simulink model "quaternion2euler"  (Simulink 10.1)
settings: Solver=VariableStepAuto  StartTime=0.0  StopTime=10.0  RelTol=1e-3  EnableMultiTasking=on
settings Model: Creator=mgreiff  LastModifiedBy=martinhe
settings DataIOCC: SaveFormat=Dataset
settings DebuggingCC: UnderspecifiedInitializationDetection=Simplified  MergeDetectMultiDrivingBlocksExec=error  SFExecutionAtInitializationDiag=warning
settings HardwareCC: ProdBitPerPointer=64  ProdBitPerSizeT=64  ProdBitPerPtrDiffT=64  ProdLargestAtomicFloat=Float  ProdIntDivRoundTo=Zero  ProdEndianess=LittleEndian  ProdWordSize=64  ProdHWDeviceType=Intel->x86-64 (Windows64)
settings ModelReferenceCC: PropagateSignalLabelsOutOfModel=on
settings GRTTargetCC: CombineOutputUpdateFcns=on  GRTInterface=off

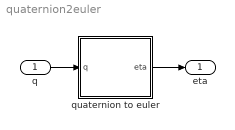
== system quaternion2euler ==
  q : Inport  PortDimensions=4
  quaternion to euler : MATLAB Function  TreatAsAtomicUnit=on
  eta : Outport  PortDimensions=3
  wires:
  q/1 -> quaternion to euler/1(q)
  quaternion to euler/1(eta) -> eta/1

== matlab function quaternion to euler ==
  data: q input double; eta output double
function eta = fcn(q)
%#codegen
phi = atan2(2*(q(1)*q(2) + q(3)*q(4)), q(1)^2 - q(2)^2 - q(3)^2 + q(4)^2);
theta = asin(2*(q(1)*q(3) - q(4)*q(2)));
psi = atan2(2*(q(1)*q(4) + q(2)*q(3)), q(1)^2 + q(2)^2 - q(3)^2 - q(4)^2);
eta = [phi;theta;psi];
